simulink model "IM_mathematical"  (R2021a)
settings: Solver=VariableStepAuto  StartTime=0.0  StopTime=2  RelTol=1e-3
values from neighbouring files (symbols this model uses):
  L1 = X1/2/pi/fs    (= 3.36819606065e-05)    [model_validation.m]    (also in rmxprt_equivalent_circuit_model.m; tf_model.m = 6.7708624294e-05)
  L2 = X2/2/pi/fs    (= 2.99288217902e-05)    [model_validation.m]    (also in rmxprt_equivalent_circuit_model.m; tf_model.m = 6.10322070604e-05)
  Lm = Xm/2/pi/fs    (= 0.000954123273506)    [model_validation.m]    (also in rmxprt_equivalent_circuit_model.m; tf_model.m = 0.0021733853742)
  R1 = 2*R1    (= 0.001579662)    [Comparison_six_three_phase.m]    (also in Untitled4.m = 3.5; Untitled7.m; enhanced_equivalent_circuit_model.m; model_validation.m = 0.000789831)
  R2 = 2*R2/0.933    (= 0.00113005359057)    [Comparison_six_three_phase.m]    (also in Untitled4.m = 4.83333333333; Untitled7.m; enhanced_equivalent_circuit_model.m; model_validation.m = 0.00052717)
  Rc = 2*Rc/0.9659    (= 45.9676985195)    [Comparison_six_three_phase.m]    (also in Untitled4.m = Vm/Ic; Untitled7.m; enhanced_equivalent_circuit_model.m; model_validation.m = 22.2001)
libraries: spsSeriesRLCBranchLib x21, spsCurrentMeasurementLib x6, spsVoltageMeasurementLib x6, spsACVoltageSourceLib x3, spsGroundLib x3, spsPowerLib x3, spsVariableResistorLib x3, simulink x1, spspowerguiLib x1
settings Model: Creator=enes_  LastModifiedBy=enes_

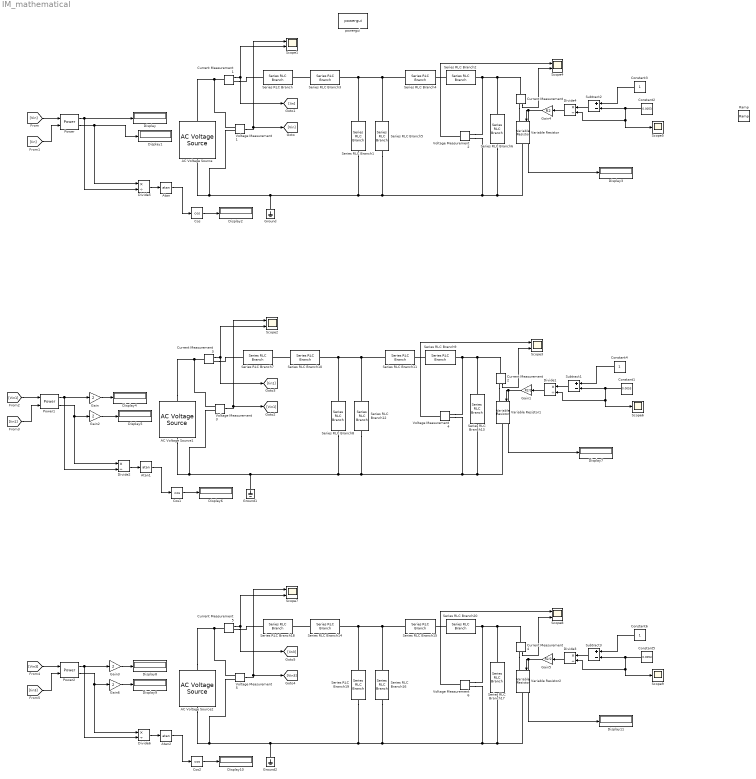
== system IM_mathematical ==
  AC Voltage Source : spsACVoltageSourceLib/AC Voltage Source  Amplitude=700*sqrt(2)*2  Phase=0  Frequency=60  SampleTime=0  Measurements=None  BusType=swing  Pref=10e3  Qref=0  Qmin=-inf  Qmax=+inf
  AC Voltage Source1 : spsACVoltageSourceLib/AC Voltage Source  Amplitude=700*sqrt(2)  Phase=0  Frequency=60  SampleTime=0  Measurements=None  BusType=swing  Pref=10e3  Qref=0  Qmin=-inf  Qmax=+inf
  AC Voltage Source2 : spsACVoltageSourceLib/AC Voltage Source  Amplitude=700*sqrt(2)  Phase=0  Frequency=60  SampleTime=0  Measurements=None  BusType=swing  Pref=10e3  Qref=0  Qmin=-inf  Qmax=+inf
  Atan : Trigonometry  Operator=atan
  Atan1 : Trigonometry  Operator=atan
  Atan2 : Trigonometry  Operator=atan
  Constant1 : Constant  Value=0.0053
  Constant2 : Constant  Value=0.0053
  Constant3 : Constant
  Constant4 : Constant
  Constant5 : Constant  Value=0.0053
  Constant6 : Constant
  Cos : Trigonometry  Operator=cos
  Cos1 : Trigonometry  Operator=cos
  Cos2 : Trigonometry  Operator=cos
  Current Measurement{,1..5} (6 alike) : spsCurrentMeasurementLib/Current Measurement  PhasorSimulation=off  OutputType=Complex  PSBequivalent=0
  Display{,1..11} (12 alike) : Display
  Divide{1..6} (6 alike) : Product  Inputs=*/
  Gain{,2..3,6} (4 alike) : Gain  Gain=2
  Gain1 : Gain  Gain=R2/2
  Gain4 : Gain  Gain=R2
  Gain5 : Gain  Gain=R2/2
  Ground : spsGroundLib/Ground  LConnTagsString=a
  Ground1 : spsGroundLib/Ground  LConnTagsString=a
  Ground2 : spsGroundLib/Ground  LConnTagsString=a
  Power : spsPowerLib/Power  Freq=60  Vinit=[1, 0]  Iinit=[1, 0]  Ts=0
      settings: SourceProductBaseCode=PS
  Power1 : spsPowerLib/Power  Freq=60  Vinit=[1, 0]  Iinit=[1, 0]  Ts=0
      settings: SourceProductBaseCode=PS
  Power2 : spsPowerLib/Power  Freq=60  Vinit=[1, 0]  Iinit=[1, 0]  Ts=0
      settings: SourceProductBaseCode=PS
  Ramp : simulink/Sources/Ramp  slope=-0.5  start=0  InitialOutput=1
  Scope{1..4,7..8} (6 alike) : Scope  NumInputPorts=2
  Scope5 : Scope
  Scope6 : Scope
  Scope9 : Scope
  Series RLC Branch : spsSeriesRLCBranchLib/Series RLC Branch  LConnTagsString=__new0  RConnTagsString=__new0  BranchType=L  Resistance=1  Inductance=L1  SetiL0=off  InitialCurrent=0  Capacitance=1e-6  Setx0=off  InitialVoltage=0  Measurements=None
  Series RLC Branch1 : spsSeriesRLCBranchLib/Series RLC Branch  LConnTagsString=__new0  RConnTagsString=__new0  BranchType=L  Resistance=1  Inductance=Lm  SetiL0=off  InitialCurrent=0  Capacitance=1e-6  Setx0=off  InitialVoltage=0  Measurements=None
  Series RLC Branch10 : spsSeriesRLCBranchLib/Series RLC Branch  LConnTagsString=__new0  RConnTagsString=__new0  BranchType=R  Resistance=R1/2  Inductance=1e-3  SetiL0=off  InitialCurrent=0  Capacitance=1e-6  Setx0=off  InitialVoltage=0  Measurements=None
  Series RLC Branch11 : spsSeriesRLCBranchLib/Series RLC Branch  LConnTagsString=__new0  RConnTagsString=__new0  BranchType=R  Resistance=R2/2  Inductance=1e-3  SetiL0=off  InitialCurrent=0  Capacitance=1e-6  Setx0=off  InitialVoltage=0  Measurements=None
  Series RLC Branch12 : spsSeriesRLCBranchLib/Series RLC Branch  LConnTagsString=__new0  RConnTagsString=__new0  BranchType=R  Resistance=Rc/2  Inductance=1e-3  SetiL0=off  InitialCurrent=0  Capacitance=1e-6  Setx0=off  InitialVoltage=0  Measurements=None
  Series RLC Branch13 : spsSeriesRLCBranchLib/Series RLC Branch  LConnTagsString=__new0  RConnTagsString=__new0  BranchType=R  Resistance=10e3  Inductance=1e-3  SetiL0=off  InitialCurrent=0  Capacitance=1e-6  Setx0=off  InitialVoltage=0  Measurements=None
  Series RLC Branch14 : spsSeriesRLCBranchLib/Series RLC Branch  LConnTagsString=__new0  RConnTagsString=__new0  BranchType=R  Resistance=R1/2  Inductance=1e-3  SetiL0=off  InitialCurrent=0  Capacitance=1e-6  Setx0=off  InitialVoltage=0  Measurements=None
  Series RLC Branch15 : spsSeriesRLCBranchLib/Series RLC Branch  LConnTagsString=__new0  RConnTagsString=__new0  BranchType=R  Resistance=R2/2  Inductance=1e-3  SetiL0=off  InitialCurrent=0  Capacitance=1e-6  Setx0=off  InitialVoltage=0  Measurements=None
  Series RLC Branch16 : spsSeriesRLCBranchLib/Series RLC Branch  LConnTagsString=__new0  RConnTagsString=__new0  BranchType=R  Resistance=Rc*0.5369  Inductance=1e-3  SetiL0=off  InitialCurrent=0  Capacitance=1e-6  Setx0=off  InitialVoltage=0  Measurements=None
  Series RLC Branch17 : spsSeriesRLCBranchLib/Series RLC Branch  LConnTagsString=__new0  RConnTagsString=__new0  BranchType=R  Resistance=10e3  Inductance=1e-3  SetiL0=off  InitialCurrent=0  Capacitance=1e-6  Setx0=off  InitialVoltage=0  Measurements=None
  Series RLC Branch18 : spsSeriesRLCBranchLib/Series RLC Branch  LConnTagsString=__new0  RConnTagsString=__new0  BranchType=L  Resistance=1  Inductance=L1/2  SetiL0=off  InitialCurrent=0  Capacitance=1e-6  Setx0=off  InitialVoltage=0  Measurements=None
  Series RLC Branch19 : spsSeriesRLCBranchLib/Series RLC Branch  LConnTagsString=__new0  RConnTagsString=__new0  BranchType=L  Resistance=1  Inductance=Lm*0.5369  SetiL0=off  InitialCurrent=0  Capacitance=1e-6  Setx0=off  InitialVoltage=0  Measurements=None
  Series RLC Branch2 : spsSeriesRLCBranchLib/Series RLC Branch  LConnTagsString=__new0  RConnTagsString=__new0  BranchType=L  Resistance=1  Inductance=L2  SetiL0=off  InitialCurrent=0  Capacitance=1e-6  Setx0=off  InitialVoltage=0  Measurements=None
  Series RLC Branch20 : spsSeriesRLCBranchLib/Series RLC Branch  LConnTagsString=__new0  RConnTagsString=__new0  BranchType=L  Resistance=1  Inductance=L2/2  SetiL0=off  InitialCurrent=0  Capacitance=1e-6  Setx0=off  InitialVoltage=0  Measurements=None
  Series RLC Branch3 : spsSeriesRLCBranchLib/Series RLC Branch  LConnTagsString=__new0  RConnTagsString=__new0  BranchType=R  Resistance=R1  Inductance=1e-3  SetiL0=off  InitialCurrent=0  Capacitance=1e-6  Setx0=off  InitialVoltage=0  Measurements=None
  Series RLC Branch4 : spsSeriesRLCBranchLib/Series RLC Branch  LConnTagsString=__new0  RConnTagsString=__new0  BranchType=R  Resistance=R2  Inductance=1e-3  SetiL0=off  InitialCurrent=0  Capacitance=1e-6  Setx0=off  InitialVoltage=0  Measurements=None
  Series RLC Branch5 : spsSeriesRLCBranchLib/Series RLC Branch  LConnTagsString=__new0  RConnTagsString=__new0  BranchType=R  Resistance=Rc  Inductance=1e-3  SetiL0=off  InitialCurrent=0  Capacitance=1e-6  Setx0=off  InitialVoltage=0  Measurements=None
  Series RLC Branch6 : spsSeriesRLCBranchLib/Series RLC Branch  LConnTagsString=__new0  RConnTagsString=__new0  BranchType=R  Resistance=10e3  Inductance=1e-3  SetiL0=off  InitialCurrent=0  Capacitance=1e-6  Setx0=off  InitialVoltage=0  Measurements=None
  Series RLC Branch7 : spsSeriesRLCBranchLib/Series RLC Branch  LConnTagsString=__new0  RConnTagsString=__new0  BranchType=L  Resistance=1  Inductance=L1/2  SetiL0=off  InitialCurrent=0  Capacitance=1e-6  Setx0=off  InitialVoltage=0  Measurements=None
  Series RLC Branch8 : spsSeriesRLCBranchLib/Series RLC Branch  LConnTagsString=__new0  RConnTagsString=__new0  BranchType=L  Resistance=1  Inductance=Lm/2  SetiL0=off  InitialCurrent=0  Capacitance=1e-6  Setx0=off  InitialVoltage=0  Measurements=None
  Series RLC Branch9 : spsSeriesRLCBranchLib/Series RLC Branch  LConnTagsString=__new0  RConnTagsString=__new0  BranchType=L  Resistance=1  Inductance=L2/2  SetiL0=off  InitialCurrent=0  Capacitance=1e-6  Setx0=off  InitialVoltage=0  Measurements=None
  Subtract1 : Sum  Inputs=+-
  Subtract2 : Sum  Inputs=+-
  Subtract3 : Sum  Inputs=+-
  Variable Resistor : spsVariableResistorLib/Variable Resistor  Rabsmin=1e-3
      settings: SourceProductBaseCode=PS
  Variable Resistor1 : spsVariableResistorLib/Variable Resistor  Rabsmin=1e-3
      settings: SourceProductBaseCode=PS
  Variable Resistor2 : spsVariableResistorLib/Variable Resistor  Rabsmin=1e-3
      settings: SourceProductBaseCode=PS
  Voltage Measurement{1..6} (6 alike) : spsVoltageMeasurementLib/Voltage Measurement  PhasorSimulation=off  OutputType=Complex  PSBequivalent=0
  powergui : spspowerguiLib/powergui  Priority=1  SimulationMode=Discrete  SampleTime=5e-6  frequency=60  Iterations=50  frequencyindice=60  Pbase=100e6  ErrMax=1e-4  UnitsV=kV  UnitsW=MW  buscounter=0  FunctionMessages=off  echomessages=off  EnableUseOfTLC=off  CurrentSourceSwitches=off  DisableSnubberDevices=off  DisableRonSwitches=off  DisableVfSwitches=off  DisplayEquations=off  AutomaticDiscreteSolvers=off  SolverType=Tustin/Backward Euler (TBE)  Interpol=off  ExternalGateDelay=off  methode=off  Ts=100  x0status=blocks  SPID=on  SwTol=0  HookPort=off  NonlinearTolerance=1e-4  nMaxIteration=100  ContinueOnMaxIteration=off  RestoreLinks=warning  ResistiveCurrentMeasurement=off  Frange=[0:2:500]  Ylog=off  Xlog=on  ShowGrid=off  save=off  variable=ZData  structure=0  ZoomFFT=off  StartTime=0.0  cycles=1  DisplayStyle=1  fundamental=60  FreqAxis=off  MaxFrequency=1000  frequencyindicesteady=1  RmsSteady=1  display=off
  wires:
  Current Measurement1/1 -> Scope1/2, [Iin]
  Constant3/1 -> Subtract2/1
  Subtract2/1 -> Divide4/1
  Divide4/1 -> Gain4/1
  Current Measurement/1 -> Scope4/2
  Voltage Measurement2/1 -> Scope4/1
  Constant2/1 -> Divide4/2, Scope5/1, Subtract2/2
  Voltage Measurement1/1 -> [Vin], Scope1/1
  [Vin] -> Power/1
  [Iin] -> Power/2
  Power/1 -> Display/1, Divide5/2
  Power/2 -> Display1/1, Divide5/1
  Divide5/1 -> Atan/1
  Atan/1 -> Cos/1
  Cos/1 -> Display2/1
  Gain4/1 -> Display3/1, Variable Resistor/1
  Divide2/1 -> Atan1/1
  [Iin1] -> Power1/2
  Atan1/1 -> Cos1/1
  Constant4/1 -> Subtract1/1
  [Vin1] -> Power1/1
  Power1/1 -> Gain/1, Divide2/2
  Gain1/1 -> Display7/1, Variable Resistor1/1
  Divide1/1 -> Gain1/1
  Current Measurement2/1 -> Scope3/2
  Cos1/1 -> Display6/1
  Current Measurement3/1 -> Scope2/2, [Iin1]
  Voltage Measurement4/1 -> Scope3/1
  Voltage Measurement3/1 -> [Vin1], Scope2/1
  Subtract1/1 -> Divide1/1
  Power1/2 -> Gain2/1, Divide2/1
  Constant1/1 -> Divide1/2, Scope6/1, Subtract1/2
  Gain/1 -> Display4/1
  Gain2/1 -> Display5/1
  Gain3/1 -> Display8/1
  Constant5/1 -> Divide3/2, Scope9/1, Subtract3/2
  Power2/2 -> Gain6/1, Divide6/1
  Cos2/1 -> Display10/1
  Constant6/1 -> Subtract3/1
  Power2/1 -> Gain3/1, Divide6/2
  [Vin3] -> Power2/1
  Divide3/1 -> Gain5/1
  [Iin3] -> Power2/2
  Gain5/1 -> Display11/1, Variable Resistor2/1
  Divide6/1 -> Atan2/1
  Voltage Measurement6/1 -> Scope8/1
  Atan2/1 -> Cos2/1
  Subtract3/1 -> Divide3/1
  Current Measurement4/1 -> Scope8/2
  Voltage Measurement5/1 -> [Vin3], Scope7/1
  Current Measurement5/1 -> Scope7/2, [Iin3]
  Gain6/1 -> Display9/1
  connections:
  Series RLC Branch3/LConn1 -- Series RLC Branch/RConn1
  Series RLC Branch4/RConn1 -- Series RLC Branch2/RConn1
  Series RLC Branch4/LConn1 -- Series RLC Branch5/LConn1 -- Series RLC Branch1/LConn1 -- Series RLC Branch3/RConn1
  Series RLC Branch2/LConn1 -- Current Measurement/LConn1 -- Series RLC Branch6/LConn1 -- Voltage Measurement2/LConn1
  Series RLC Branch1/RConn1 -- Variable Resistor/RConn1 -- Series RLC Branch6/RConn1 -- Voltage Measurement2/LConn2 -- Series RLC Branch5/RConn1 -- Voltage Measurement1/LConn2 -- AC Voltage Source/LConn1 -- Ground/LConn1
  Current Measurement/RConn1 -- Variable Resistor/LConn1
  Voltage Measurement1/LConn1 -- Current Measurement1/LConn1 -- AC Voltage Source/RConn1
  Current Measurement1/RConn1 -- Series RLC Branch/LConn1
  Voltage Measurement4/LConn2 -- Variable Resistor1/RConn1 -- Series RLC Branch13/RConn1 -- Series RLC Branch8/RConn1 -- Voltage Measurement3/LConn2 -- AC Voltage Source1/LConn1 -- Ground1/LConn1 -- Series RLC Branch12/RConn1
  Series RLC Branch13/LConn1 -- Voltage Measurement4/LConn1 -- Series RLC Branch9/LConn1 -- Current Measurement2/LConn1
  Series RLC Branch10/RConn1 -- Series RLC Branch8/LConn1 -- Series RLC Branch11/LConn1 -- Series RLC Branch12/LConn1
  AC Voltage Source1/RConn1 -- Voltage Measurement3/LConn1 -- Current Measurement3/LConn1
  Current Measurement2/RConn1 -- Variable Resistor1/LConn1
  Current Measurement3/RConn1 -- Series RLC Branch7/LConn1
  Series RLC Branch10/LConn1 -- Series RLC Branch7/RConn1
  Series RLC Branch11/RConn1 -- Series RLC Branch9/RConn1
  Voltage Measurement6/LConn2 -- Variable Resistor2/RConn1 -- Series RLC Branch17/RConn1 -- Series RLC Branch16/RConn1 -- Series RLC Branch19/RConn1 -- Ground2/LConn1 -- Voltage Measurement5/LConn2 -- AC Voltage Source2/LConn1
  Series RLC Branch16/LConn1 -- Series RLC Branch15/LConn1 -- Series RLC Branch19/LConn1 -- Series RLC Branch14/RConn1
  Series RLC Branch17/LConn1 -- Current Measurement4/LConn1 -- Voltage Measurement6/LConn1 -- Series RLC Branch20/LConn1
  AC Voltage Source2/RConn1 -- Voltage Measurement5/LConn1 -- Current Measurement5/LConn1
  Current Measurement4/RConn1 -- Variable Resistor2/LConn1
  Series RLC Branch14/LConn1 -- Series RLC Branch18/RConn1
  Current Measurement5/RConn1 -- Series RLC Branch18/LConn1
  Series RLC Branch15/RConn1 -- Series RLC Branch20/RConn1
